simulink model "QuadCopter_2"  (R2018a)
settings: Solver=VariableStepAuto  StartTime=0.0  StopTime=60  MaxStep=0.1  RelTol=1e-3
values from neighbouring files (symbols this model uses):
  d = 2.4*10^-3    (= 0.0024)    [ScrValBackup.m]    (also in corke_plot.m = quad.d)
  dx0 = 0    [ScrValBackup.m]
  dy0 = 0    [ScrValBackup.m]
  dz0 = 0    [ScrValBackup.m]
  g = 9.81    [ScrValBackup.m]
  Ixx = 5.9*10-3    (= 56)    [ScrValBackup.m]    (also in quadrotorInitialValues.m)
  Iyy = 5.9*10-3    (= 56)    [ScrValBackup.m]    (also in quadrotorInitialValues.m)
  Izz = 1.16*10-3    (= 8.6)    [ScrValBackup.m]    (also in quadrotorInitialValues.m)
  K_lin = [   15.6000,    0.0000,    7.9000,    0.0000,         0 ... (first row only)    [ScrValBackup.m]
  kr = 0.1    [ScrValBackup.m]
  kt = 0.1    [ScrValBackup.m]
  l = 0.255    [ScrValBackup.m]
  m = 0.5    [ScrValBackup.m]
  p0 = 0    [ScrValBackup.m]
  phi0 = 0    [ScrValBackup.m]
  psi0 = 0.1    [ScrValBackup.m]
  q0 = 0    [ScrValBackup.m]
  r0 = 0.1177    [ScrValBackup.m]
  theta0 = 0    [ScrValBackup.m]
  x0 = 1    [ScrValBackup.m]    (also in corke_dynamics.m = init; corke_plot.m = [])
  x_coeff = A^-1*x_constr    [ScrValBackup.m]
  xd = 1    [ScrValBackup.m]
  y0 = 1    [ScrValBackup.m]
  y_coeff = A^-1*y_constr    [ScrValBackup.m]
  yd = 1    [ScrValBackup.m]
  z0 = 1    [ScrValBackup.m]
  z_coeff = A^-1*z_constr    [ScrValBackup.m]
  zd = 5    [ScrValBackup.m]
libraries: simulink x3, aerolibutil x1
settings Model: Creator=blue_orangotan  LastModifiedBy=giuseppe
settings SolverCC: ZeroCrossAlgorithm=Adaptive
settings DebuggingCC: MaxConsecutiveZCsMsg=warning  MaskedZcDiagnostic=none

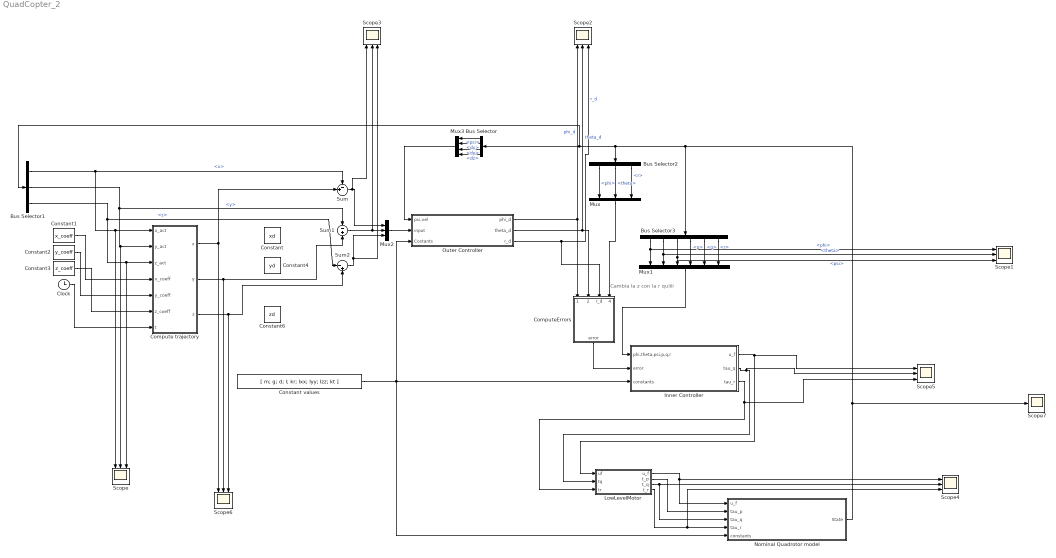
== system QuadCopter_2 ==
  note: Cambia la z con la r quiiii
  Bus Selector : BusSelector  OutputSignals=psi,dx,dy,dz
  Bus Selector1 : BusSelector  OutputSignals=x,y,z
  Bus Selector2 : BusSelector  OutputSignals=phi,theta,r
  Bus Selector3 : BusSelector  OutputSignals=phi,theta,psi,p,q,r
  Clock : Clock
  Compute trajectory : MATLAB Function  TreatAsAtomicUnit=on
  "ComputeErrors " : Subsystem
  Constant : Constant  Value=xd
  Constant values : Constant  Value=[ m; g; d; l; kr; Ixx; Iyy; Izz; kt ]
  Constant1 : Constant  Value=x_coeff
  Constant2 : Constant  Value=y_coeff
  Constant3 : Constant  Value=z_coeff
  Constant4 : Constant  Value=yd
  Constant6 : Constant  Value=zd
  "Inner Controller " : Subsystem
  LowLevelMotor : Subsystem
  Mux : Mux  Inputs=3
  Mux1 : Mux  Inputs=6
  Mux2 : Mux  Inputs=3
  Mux3 : Mux
  Nominal Quadrotor model : Subsystem
  "Outer Controller " : Subsystem
  Scope{,1..6} (7 alike) : Scope  NumInputPorts=3
  Scope7 : Scope
  Sum : Sum  Inputs=-+|
  Sum1 : Sum  Inputs=-+
  Sum2 : Sum  Inputs=|-+
  wires:
  Nominal Quadrotor model/1(State) -> Scope7/1, Bus Selector/1, Bus Selector1/1, Bus Selector2/1, Bus Selector3/1
  Constant values/1 -> "Inner Controller "/3(constants), Nominal Quadrotor model/5(constants), "Outer Controller "/3(Costants)
  Constant1/1 -> Compute trajectory/4(x_coeff)
  Constant2/1 -> Compute trajectory/5(y_coeff)
  Constant3/1 -> Compute trajectory/6(z_coeff)
  Clock/1 -> Compute trajectory/7(t)
  Bus Selector1/1 -> Sum/1, Compute trajectory/1(x_act), Scope/1  "<x>"
  Bus Selector1/2 -> Scope/2, Compute trajectory/2(y_act), Sum1/1  "<y>"
  Bus Selector1/3 -> Scope/3, Compute trajectory/3(z_act), Sum2/1  "<z>"
  "ComputeErrors "/1(error) -> "Inner Controller "/2(error)
  Bus Selector2/1 -> Mux/1  "<phi>"
  Bus Selector2/2 -> Mux/2  "<theta>"
  Bus Selector2/3 -> Mux/3  "<r>"
  Mux/1 -> "ComputeErrors "/4(Curr_values)
  Bus Selector3/1 -> Mux1/1, Scope1/1  "<phi>"
  Bus Selector3/2 -> Mux1/2, Scope1/2  "<theta>"
  Bus Selector3/3 -> Scope1/3, Mux1/3  "<psi>"
  Bus Selector3/4 -> Mux1/4  "<p>"
  Bus Selector3/5 -> Mux1/5  "<q>"
  Bus Selector3/6 -> Mux1/6  "<r>"
  Mux1/1 -> "Inner Controller "/1(phi,theta,psi,p,q,r)
  "Inner Controller "/1(u_f) -> Scope5/1, LowLevelMotor/1(uf)
  "Inner Controller "/2(tau_q) -> Scope5/2, LowLevelMotor/2("tq ")
  "Inner Controller "/3(tau_r) -> Scope5/3, LowLevelMotor/3(tr)
  LowLevelMotor/1(u_f) -> Scope4/1, Nominal Quadrotor model/1(u_f)
  LowLevelMotor/2(t_p) -> Nominal Quadrotor model/2(tau_p)
  LowLevelMotor/3(t_q) -> Scope4/2, Nominal Quadrotor model/3(tau_q)
  LowLevelMotor/4(t_r) -> Scope4/3, Nominal Quadrotor model/4(tau_r)
  "Outer Controller "/1("phi_d ") -> "ComputeErrors "/1(phi_d), Scope2/1  "phi_d"
  "Outer Controller "/2(theta_d) -> "ComputeErrors "/2(theta_d), Scope2/2  "theta_d"
  Sum/1 -> Scope3/1, Mux2/1
  Sum1/1 -> Mux2/2, Scope3/2
  Sum2/1 -> Scope3/3, Mux2/3
  Mux2/1 -> "Outer Controller "/2(input)
  "Outer Controller "/3(r_d) -> "ComputeErrors "/3(r_d), Scope2/3  "r_d"
  Compute trajectory/2(y) -> Sum1/2, Scope6/2
  Compute trajectory/1(x) -> Sum/2, Scope6/1
  Compute trajectory/3(z) -> Sum2/2, Scope6/3
  Bus Selector/1 -> Mux3/1  "<psi>"
  Bus Selector/2 -> Mux3/2  "<dx>"
  Bus Selector/3 -> Mux3/3  "<dy>"
  Bus Selector/4 -> Mux3/4  "<dz>"
  Mux3/1 -> "Outer Controller "/1(psi,vel)

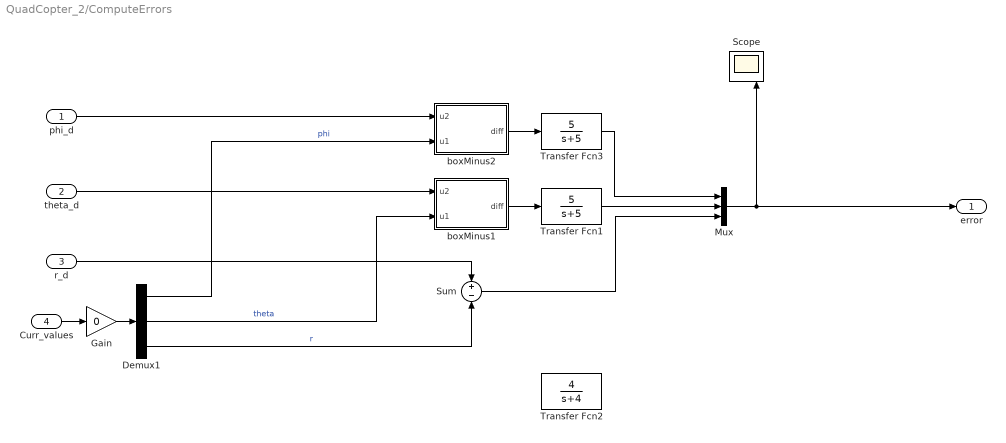
== system QuadCopter_2/ComputeErrors  ==
  phi_d : Inport
  theta_d : Inport  Port=2
  r_d : Inport  Port=3
  Curr_values : Inport  Port=4
  Demux1 : Demux  Outputs=3
  Gain : Gain  Gain=0
  Mux : Mux  Inputs=3
  Scope : Scope  NumInputPorts=3
  Sum : Sum  Inputs=+-
  Transfer Fcn1 : TransferFcn  Numerator=[5]  Denominator=[1 5]
  Transfer Fcn2 : TransferFcn  Numerator=[4]  Denominator=[1 4]
  Transfer Fcn3 : TransferFcn  Numerator=[5]  Denominator=[1 5]
  boxMinus1 : MATLAB Function  TreatAsAtomicUnit=on
  boxMinus2 : MATLAB Function  TreatAsAtomicUnit=on
  error : Outport
  wires:
  phi_d/1 -> boxMinus2/1(u2)
  Demux1/1 -> boxMinus2/2(u1)  "phi"
  theta_d/1 -> boxMinus1/1(u2)
  Demux1/2 -> boxMinus1/2(u1)  "theta"
  r_d/1 -> Sum/1
  Demux1/3 -> Sum/2  "r"
  Mux/1 -> error/1, Scope/3
  Sum/1 -> Mux/3
  boxMinus2/1(diff) -> Transfer Fcn3/1
  boxMinus1/1(diff) -> Transfer Fcn1/1
  Transfer Fcn3/1 -> Mux/1
  Transfer Fcn1/1 -> Mux/2
  Curr_values/1 -> Gain/1
  Gain/1 -> Demux1/1

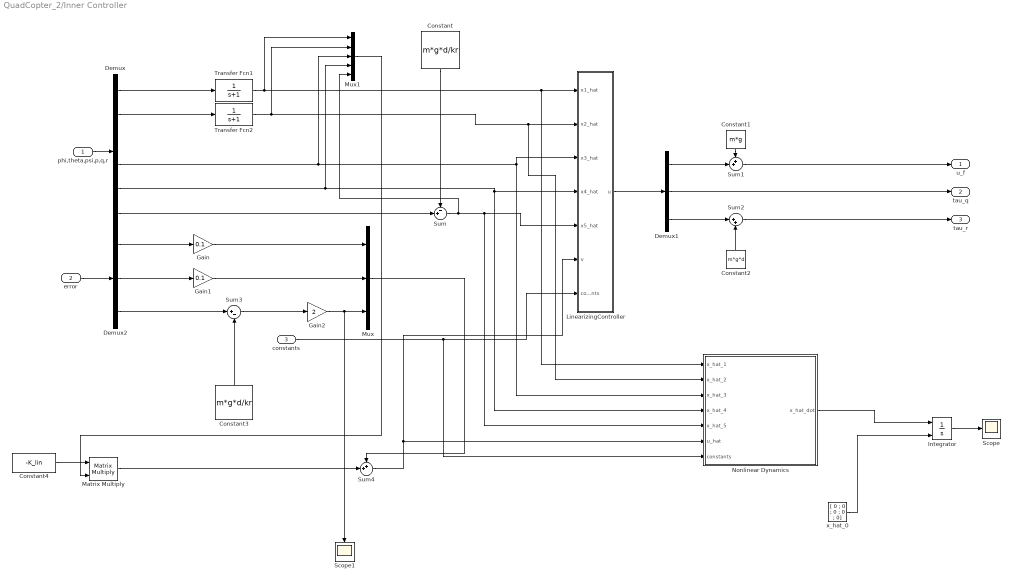
== system QuadCopter_2/Inner Controller  ==
  phi,theta,psi,p,q,r : Inport
  error : Inport  Port=2
  constants : Inport  Port=3
  Constant : Constant  Value=m*g*d/kr
  Constant1 : Constant  Value=m*g
  Constant2 : Constant  Value=m*g*d
  Constant3 : Constant  Value=m*g*d/kr
  Constant4 : Constant  Value=-K_lin
  Demux : Demux  Outputs=6
  Demux1 : Demux  Outputs=3
  Demux2 : Demux  Outputs=3
  Gain : Gain  Gain=0.1
  Gain1 : Gain  Gain=0.1
  Gain2 : Gain  Gain=2
  Integrator : Integrator  InitialConditionSource=external
  LinearizingController : MATLAB Function  TreatAsAtomicUnit=on
  Matrix Multiply : Product  Multiplication=Matrix(*)
  Mux : Mux  Inputs=3
  Mux1 : Mux  Inputs=5
  "Nonlinear Dynamics " : MATLAB Function  TreatAsAtomicUnit=on
  Scope : Scope
  Scope1 : Scope
  Sum : Sum  Inputs=-+|
  Sum1 : Sum  Inputs=++|
  Sum2 : Sum  Inputs=|++
  Sum3 : Sum  Inputs=|+-
  Sum4 : Sum  Inputs=++|
  Transfer Fcn1 : TransferFcn  Denominator=[1 1]
  Transfer Fcn2 : TransferFcn  Denominator=[1 1]
  x_hat_0 : Constant  Value=[ 0 ; 0 ; 0 ; 0 ; 0]
  u_f : Outport
  tau_q : Outport  Port=2
  tau_r : Outport  Port=3
  wires:
  phi,theta,psi,p,q,r/1 -> Demux/1
  Demux/1 -> Transfer Fcn1/1
  Demux/2 -> Transfer Fcn2/1
  Demux/4 -> Mux1/3, LinearizingController/3(x3_hat), "Nonlinear Dynamics "/3(x_hat_3)
  Demux/5 -> Mux1/4, "Nonlinear Dynamics "/4(x_hat_4), LinearizingController/4(x4_hat)
  "Nonlinear Dynamics "/1(x_hat_dot) -> Integrator/1
  x_hat_0/1 -> Integrator/2
  Constant/1 -> Sum/1
  Sum/1 -> Mux1/5, "Nonlinear Dynamics "/5(x_hat_5), LinearizingController/5(x5_hat)
  Demux1/3 -> Sum2/1
  Demux1/1 -> Sum1/2
  Constant1/1 -> Sum1/1
  Sum1/1 -> u_f/1
  Demux1/2 -> tau_q/1
  Constant2/1 -> Sum2/2
  Sum2/1 -> tau_r/1
  LinearizingController/1(u) -> Demux1/1
  Integrator/1 -> Scope/1
  constants/1 -> "Nonlinear Dynamics "/7(constants), LinearizingController/7(constants)
  Demux/6 -> Sum/2
  error/1 -> Demux2/1
  Constant3/1 -> Sum3/2
  Sum3/1 -> Gain2/1
  Transfer Fcn1/1 -> Mux1/1, "Nonlinear Dynamics "/1(x_hat_1), LinearizingController/1(x1_hat)
  Transfer Fcn2/1 -> Mux1/2, "Nonlinear Dynamics "/2(x_hat_2), LinearizingController/2(x2_hat)
  Demux2/1 -> Gain/1
  Demux2/2 -> Gain1/1
  Constant4/1 -> Matrix Multiply/1
  Mux1/1 -> Matrix Multiply/2
  Matrix Multiply/1 -> Sum4/2
  Mux/1 -> Sum4/1
  Sum4/1 -> "Nonlinear Dynamics "/6(u_hat), LinearizingController/6(v)
  Gain/1 -> Mux/1
  Gain1/1 -> Mux/2
  Demux2/3 -> Sum3/1
  Gain2/1 -> Mux/3, Scope1/1

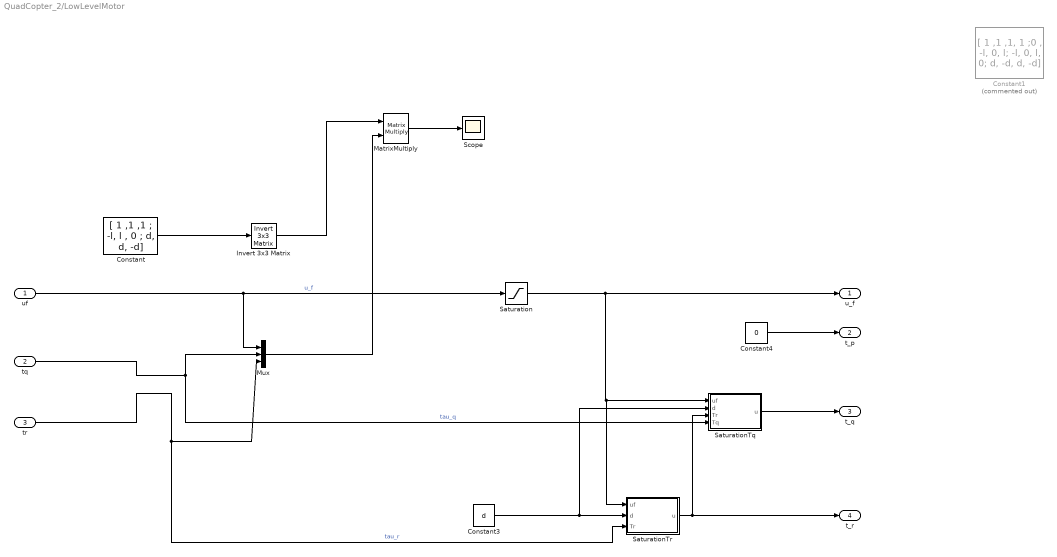
== system QuadCopter_2/LowLevelMotor ==
  uf : Inport
  "tq " : Inport  Port=2
  tr : Inport  Port=3
  Constant : Constant  Value=[ 1 ,1 ,1 ; -l, l , 0 ; d, d, -d]
  Constant1 : Constant  Commented=on  Value="[ 1 ,1 ,1, 1 ;0 , -l, 0, l;  -l, 0, l, 0; d, -d, d, -d]"
  Constant3 : Constant  Value=d
  Constant4 : Constant  Value=0
  Invert 3x3 Matrix : aerolibutil/Invert  3x3 Matrix
  MatrixMultiply : Product  Multiplication=Matrix(*)
  Mux : Mux  Inputs=3
  Saturation : Saturate  UpperLimit=15
  SaturationTq : MATLAB Function  TreatAsAtomicUnit=on
  SaturationTr : MATLAB Function  TreatAsAtomicUnit=on
  Scope : Scope
  u_f : Outport
  t_p : Outport  Port=2
  t_q : Outport  Port=3
  t_r : Outport  Port=4
  wires:
  "tq "/1 -> SaturationTq/4(Tq), Mux/2  "tau_q"
  tr/1 -> Mux/3, SaturationTr/3(Tr)  "tau_r"
  uf/1 -> Mux/1, Saturation/1  "u_f"
  Constant/1 -> Invert 3x3 Matrix/1
  Constant4/1 -> t_p/1
  Constant3/1 -> SaturationTq/2(d), SaturationTr/2(d)
  SaturationTr/1(u) -> SaturationTq/3(Tr), t_r/1
  SaturationTq/1(u) -> t_q/1
  Invert 3x3 Matrix/1 -> MatrixMultiply/1
  Saturation/1 -> SaturationTr/1(uf), SaturationTq/1(uf), u_f/1
  Mux/1 -> MatrixMultiply/2
  MatrixMultiply/1 -> Scope/1

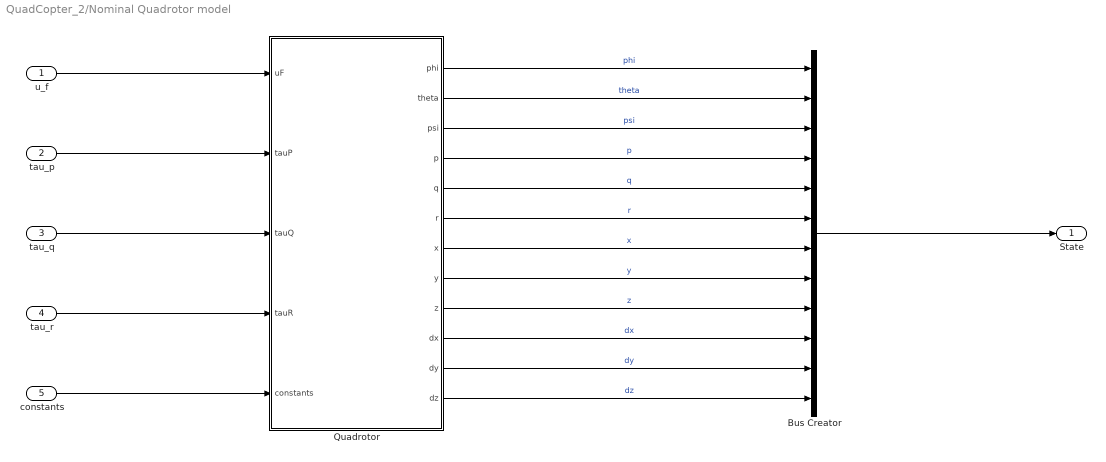
== system QuadCopter_2/Nominal Quadrotor model ==
  u_f : Inport
  tau_p : Inport  Port=2
  tau_q : Inport  Port=3
  tau_r : Inport  Port=4
  constants : Inport  Port=5
  Bus Creator : BusCreator  Inputs=12
  "Quadrotor " : Subsystem
  State : Outport
  wires:
  u_f/1 -> "Quadrotor "/1(uF)
  tau_q/1 -> "Quadrotor "/3(tauQ)
  tau_r/1 -> "Quadrotor "/4(tauR)
  constants/1 -> "Quadrotor "/5(constants)
  tau_p/1 -> "Quadrotor "/2(tauP)
  "Quadrotor "/1(phi) -> Bus Creator/1  "phi"
  "Quadrotor "/2(theta) -> Bus Creator/2  "theta"
  "Quadrotor "/3(psi) -> Bus Creator/3  "psi"
  "Quadrotor "/4(p) -> Bus Creator/4  "p"
  "Quadrotor "/5(q) -> Bus Creator/5  "q"
  "Quadrotor "/6(r) -> Bus Creator/6  "r"
  "Quadrotor "/7(x) -> Bus Creator/7  "x"
  "Quadrotor "/8(y) -> Bus Creator/8  "y"
  "Quadrotor "/9(z) -> Bus Creator/9  "z"
  Bus Creator/1 -> State/1
  "Quadrotor "/10(dx) -> Bus Creator/10  "dx"
  "Quadrotor "/11(dy) -> Bus Creator/11  "dy"
  "Quadrotor "/12(dz) -> Bus Creator/12  "dz"

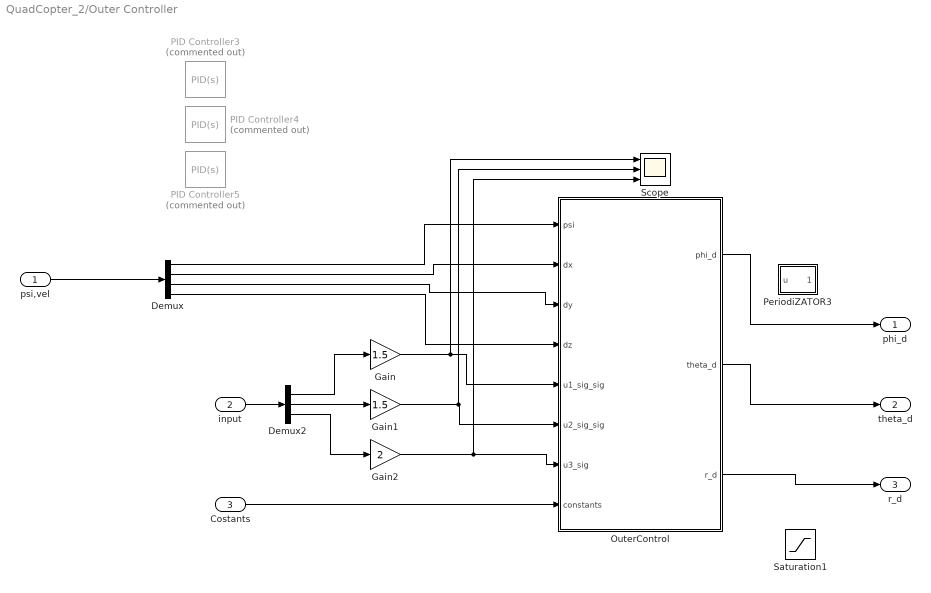
== system QuadCopter_2/Outer Controller  ==
  psi,vel : Inport  SampleTime=0.1
  input : Inport  Port=2
  Costants : Inport  Port=3
  Demux : Demux
  Demux2 : Demux  Outputs=3
  Gain : Gain  Gain=1.5
  Gain1 : Gain  Gain=1.5
  Gain2 : Gain  Gain=2
  OuterControl : MATLAB Function  TreatAsAtomicUnit=on
  PID Controller3 : simulink/Continuous/PID Controller  Commented=on  Controller=PID  TimeDomain=Continuous-time  SampleTime=-1  IntegratorMethod=Forward Euler  FilterMethod=Forward Euler  Form=Parallel  UseFilter=on  ControllerParametersSource=internal  P=-3.31812549008861e-05  I=-2.04327645124417e-11  D=-11.9723513961423  N=0.0120629646409386  InitialConditionSource=internal  InitialConditionForIntegrator=0  InitialConditionForFilter=0  ExternalReset=none  LimitOutput=off  UpperSaturationLimit=inf  LowerSaturationLimit=-inf  LinearizeAsGain=on  AntiWindupMode=none  Kb=1  TrackingMode=off  Kt=1  PParamMin=[]  PParamMax=[]  IParamMin=[]  IParamMax=[]  DParamMin=[]  DParamMax=[]  NParamMin=[]  NParamMax=[]  KbParamMin=[]  KbParamMax=[]  KtParamMin=[]  KtParamMax=[]  POutMin=[]  POutMax=[]  IOutMin=[]  IOutMax=[]  DOutMin=[]  DOutMax=[]  NOutMin=[]  NOutMax=[]  KbOutMin=[]  KbOutMax=[]  KtOutMin=[]  KtOutMax=[]  IntegratorOutMin=[]  IntegratorOutMax=[]  FilterOutMin=[]  FilterOutMax=[]  SumOutMin=[]  SumOutMax=[]  SumI1OutMin=[]  SumI1OutMax=[]  SumI2OutMin=[]  SumI2OutMax=[]  SumI3OutMin=[]  SumI3OutMax=[]  SumDOutMin=[]  SumDOutMax=[]  SaturationOutMin=[]  SaturationOutMax=[]  IntegratorContinuousStateAttributes=''  IntegratorStateMustResolveToSignalObject=off  IntegratorRTWStateStorageClass=Auto  FilterContinuousStateAttributes=''  FilterStateMustResolveToSignalObject=off  FilterRTWStateStorageClass=Auto  DifferentiatorICPrevScaledInput=0  DifferentiatorOutMin=[]  DifferentiatorOutMax=[]  FilterDiffOutCoefMin=[]  FilterDiffOutCoefMax=[]  SumDenOutMin=[]  SumDenOutMax=[]  SumNumOutMin=[]  SumNumOutMax=[]  ReciprocalOutMin=[]  ReciprocalOutMax=[]  DivideOutMin=[]  DivideOutMax=[]  TunerSelectOption=Transfer Function Based (PID Tuner App)
  PID Controller4 : simulink/Continuous/PID Controller  Commented=on  Controller=PID  TimeDomain=Continuous-time  SampleTime=-1  IntegratorMethod=Forward Euler  FilterMethod=Forward Euler  Form=Parallel  UseFilter=on  ControllerParametersSource=internal  P=-3.31812549008861e-05  I=-2.04327645124417e-11  D=-11.9723513961423  N=0.0120629646409386  InitialConditionSource=internal  InitialConditionForIntegrator=0  InitialConditionForFilter=0  ExternalReset=none  LimitOutput=off  UpperSaturationLimit=inf  LowerSaturationLimit=-inf  LinearizeAsGain=on  AntiWindupMode=none  Kb=1  TrackingMode=off  Kt=1  PParamMin=[]  PParamMax=[]  IParamMin=[]  IParamMax=[]  DParamMin=[]  DParamMax=[]  NParamMin=[]  NParamMax=[]  KbParamMin=[]  KbParamMax=[]  KtParamMin=[]  KtParamMax=[]  POutMin=[]  POutMax=[]  IOutMin=[]  IOutMax=[]  DOutMin=[]  DOutMax=[]  NOutMin=[]  NOutMax=[]  KbOutMin=[]  KbOutMax=[]  KtOutMin=[]  KtOutMax=[]  IntegratorOutMin=[]  IntegratorOutMax=[]  FilterOutMin=[]  FilterOutMax=[]  SumOutMin=[]  SumOutMax=[]  SumI1OutMin=[]  SumI1OutMax=[]  SumI2OutMin=[]  SumI2OutMax=[]  SumI3OutMin=[]  SumI3OutMax=[]  SumDOutMin=[]  SumDOutMax=[]  SaturationOutMin=[]  SaturationOutMax=[]  IntegratorContinuousStateAttributes=''  IntegratorStateMustResolveToSignalObject=off  IntegratorRTWStateStorageClass=Auto  FilterContinuousStateAttributes=''  FilterStateMustResolveToSignalObject=off  FilterRTWStateStorageClass=Auto  DifferentiatorICPrevScaledInput=0  DifferentiatorOutMin=[]  DifferentiatorOutMax=[]  FilterDiffOutCoefMin=[]  FilterDiffOutCoefMax=[]  SumDenOutMin=[]  SumDenOutMax=[]  SumNumOutMin=[]  SumNumOutMax=[]  ReciprocalOutMin=[]  ReciprocalOutMax=[]  DivideOutMin=[]  DivideOutMax=[]  TunerSelectOption=Transfer Function Based (PID Tuner App)
  PID Controller5 : simulink/Continuous/PID Controller  Commented=on  Controller=PID  TimeDomain=Continuous-time  SampleTime=-1  IntegratorMethod=Forward Euler  FilterMethod=Forward Euler  Form=Parallel  UseFilter=on  ControllerParametersSource=internal  P=-3.31812549008861e-05  I=-2.04327645124417e-11  D=-11.9723513961423  N=0.0120629646409386  InitialConditionSource=internal  InitialConditionForIntegrator=0  InitialConditionForFilter=0  ExternalReset=none  LimitOutput=off  UpperSaturationLimit=inf  LowerSaturationLimit=-inf  LinearizeAsGain=on  AntiWindupMode=none  Kb=1  TrackingMode=off  Kt=1  PParamMin=[]  PParamMax=[]  IParamMin=[]  IParamMax=[]  DParamMin=[]  DParamMax=[]  NParamMin=[]  NParamMax=[]  KbParamMin=[]  KbParamMax=[]  KtParamMin=[]  KtParamMax=[]  POutMin=[]  POutMax=[]  IOutMin=[]  IOutMax=[]  DOutMin=[]  DOutMax=[]  NOutMin=[]  NOutMax=[]  KbOutMin=[]  KbOutMax=[]  KtOutMin=[]  KtOutMax=[]  IntegratorOutMin=[]  IntegratorOutMax=[]  FilterOutMin=[]  FilterOutMax=[]  SumOutMin=[]  SumOutMax=[]  SumI1OutMin=[]  SumI1OutMax=[]  SumI2OutMin=[]  SumI2OutMax=[]  SumI3OutMin=[]  SumI3OutMax=[]  SumDOutMin=[]  SumDOutMax=[]  SaturationOutMin=[]  SaturationOutMax=[]  IntegratorContinuousStateAttributes=''  IntegratorStateMustResolveToSignalObject=off  IntegratorRTWStateStorageClass=Auto  FilterContinuousStateAttributes=''  FilterStateMustResolveToSignalObject=off  FilterRTWStateStorageClass=Auto  DifferentiatorICPrevScaledInput=0  DifferentiatorOutMin=[]  DifferentiatorOutMax=[]  FilterDiffOutCoefMin=[]  FilterDiffOutCoefMax=[]  SumDenOutMin=[]  SumDenOutMax=[]  SumNumOutMin=[]  SumNumOutMax=[]  ReciprocalOutMin=[]  ReciprocalOutMax=[]  DivideOutMin=[]  DivideOutMax=[]  TunerSelectOption=Transfer Function Based (PID Tuner App)
  PeriodiZATOR3 : MATLAB Function  TreatAsAtomicUnit=on
  Saturation1 : Saturate  UpperLimit=5  LowerLimit=0
  Scope : Scope  NumInputPorts=3
  "phi_d " : Outport
  theta_d : Outport  Port=2
  r_d : Outport  Port=3
  wires:
  Costants/1 -> OuterControl/8(constants)
  input/1 -> Demux2/1
  OuterControl/3(r_d) -> r_d/1
  Demux2/1 -> Gain/1
  Demux2/2 -> Gain1/1
  Demux2/3 -> Gain2/1
  Gain/1 -> Scope/1, OuterControl/5(u1_sig_sig)
  Gain1/1 -> Scope/2, OuterControl/6(u2_sig_sig)
  Gain2/1 -> Scope/3, OuterControl/7(u3_sig)
  OuterControl/1(phi_d) -> "phi_d "/1
  OuterControl/2(theta_d) -> theta_d/1
  psi,vel/1 -> Demux/1
  Demux/1 -> OuterControl/1(psi)
  Demux/2 -> OuterControl/2(dx)
  Demux/3 -> OuterControl/3(dy)
  Demux/4 -> OuterControl/4(dz)

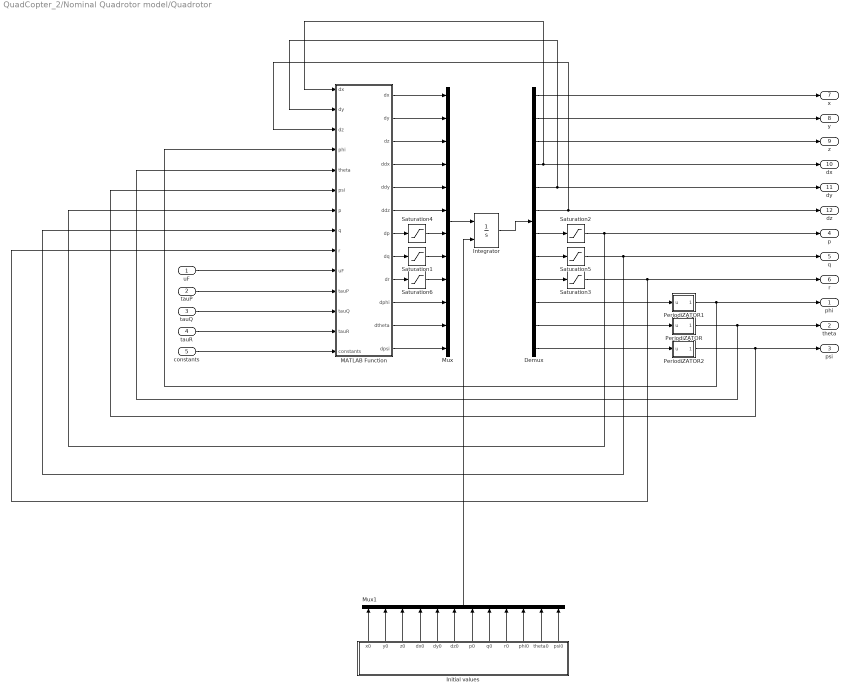
== system QuadCopter_2/Nominal Quadrotor model/Quadrotor  ==
  uF : Inport
  tauP : Inport  Port=2
  tauQ : Inport  Port=3
  tauR : Inport  Port=4
  constants : Inport  Port=5
  Demux : Demux  Outputs=12
  "Initial values " : Subsystem
  Integrator : Integrator  InitialConditionSource=external
  MATLAB Function : MATLAB Function  TreatAsAtomicUnit=on
  Mux : Mux  Inputs=12
  Mux1 : Mux  Inputs=12
  PeriodiZATOR : MATLAB Function  TreatAsAtomicUnit=on
  PeriodiZATOR1 : MATLAB Function  TreatAsAtomicUnit=on
  PeriodiZATOR2 : MATLAB Function  TreatAsAtomicUnit=on
  Saturation1 : Saturate
  Saturation2 : Saturate  UpperLimit=4  LowerLimit=-4
  Saturation3 : Saturate  UpperLimit=6  LowerLimit=0
  Saturation4 : Saturate
  Saturation5 : Saturate  UpperLimit=4  LowerLimit=-4
  Saturation6 : Saturate
  phi : Outport
  theta : Outport  Port=2
  psi : Outport  Port=3
  p : Outport  Port=4
  q : Outport  Port=5
  r : Outport  Port=6
  x : Outport  Port=7
  y : Outport  Port=8
  z : Outport  Port=9
  dx : Outport  Port=10
  dy : Outport  Port=11
  dz : Outport  Port=12
  wires:
  uF/1 -> MATLAB Function/10(uF)
  tauP/1 -> MATLAB Function/11(tauP)
  tauQ/1 -> MATLAB Function/12(tauQ)
  tauR/1 -> MATLAB Function/13(tauR)
  PeriodiZATOR/1(angle) -> MATLAB Function/5(theta), theta/1
  PeriodiZATOR1/1(angle) -> MATLAB Function/4(phi), phi/1
  PeriodiZATOR2/1(angle) -> MATLAB Function/6(psi), psi/1
  constants/1 -> MATLAB Function/14(constants)
  MATLAB Function/1(dx) -> Mux/1
  MATLAB Function/2(dy) -> Mux/2
  MATLAB Function/3(dz) -> Mux/3
  MATLAB Function/4(ddx) -> Mux/4
  MATLAB Function/5(ddy) -> Mux/5
  MATLAB Function/6(ddz) -> Mux/6
  MATLAB Function/7(dp) -> Saturation4/1
  MATLAB Function/8(dq) -> Saturation1/1
  MATLAB Function/9(dr) -> Saturation6/1
  MATLAB Function/10(dphi) -> Mux/10
  MATLAB Function/11(dtheta) -> Mux/11
  MATLAB Function/12(dpsi) -> Mux/12
  Mux/1 -> Integrator/1
  "Initial values "/1(x0) -> Mux1/1
  "Initial values "/2(y0) -> Mux1/2
  "Initial values "/3(z0) -> Mux1/3
  "Initial values "/4(dx0) -> Mux1/4
  "Initial values "/5(dy0) -> Mux1/5
  "Initial values "/6(dz0) -> Mux1/6
  "Initial values "/7(p0) -> Mux1/7
  "Initial values "/8(q0) -> Mux1/8
  "Initial values "/9(r0) -> Mux1/9
  "Initial values "/10(phi0) -> Mux1/10
  "Initial values "/11(theta0) -> Mux1/11
  "Initial values "/12(psi0) -> Mux1/12
  Mux1/1 -> Integrator/2
  Integrator/1 -> Demux/1
  Demux/1 -> x/1
  Demux/2 -> y/1
  Demux/3 -> z/1
  Demux/5 -> dy/1, MATLAB Function/2("dy ")
  Demux/6 -> dz/1, MATLAB Function/3("dz ")
  Demux/10 -> PeriodiZATOR1/1(u)
  Demux/11 -> PeriodiZATOR/1(u)
  Demux/12 -> PeriodiZATOR2/1(u)
  Demux/9 -> Saturation3/1
  Demux/7 -> Saturation2/1
  Demux/8 -> Saturation5/1
  Saturation3/1 -> r/1, MATLAB Function/9(r)
  Saturation4/1 -> Mux/7
  Saturation1/1 -> Mux/8
  Saturation2/1 -> p/1, MATLAB Function/7(p)
  Saturation5/1 -> q/1, MATLAB Function/8(q)
  Saturation6/1 -> Mux/9
  Demux/4 -> dx/1, MATLAB Function/1("dx ")

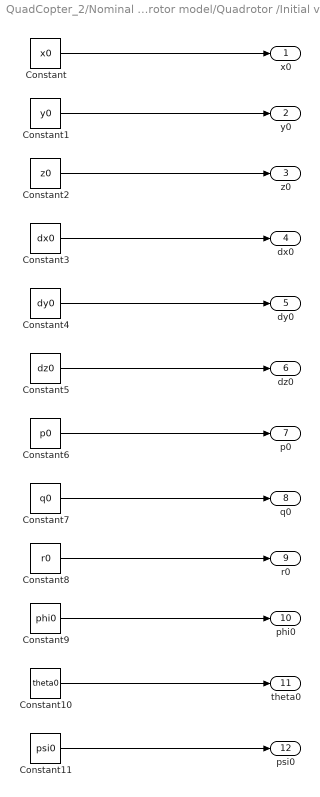
== system QuadCopter_2/Nominal Quadrotor model/Quadrotor /Initial values  ==
  Constant : Constant  Value=x0
  Constant1 : Constant  Value=y0
  Constant10 : Constant  Value=theta0
  Constant11 : Constant  Value=psi0
  Constant2 : Constant  Value=z0
  Constant3 : Constant  Value=dx0
  Constant4 : Constant  Value=dy0
  Constant5 : Constant  Value=dz0
  Constant6 : Constant  Value=p0
  Constant7 : Constant  Value=q0
  Constant8 : Constant  Value=r0
  Constant9 : Constant  Value=phi0
  x0 : Outport
  y0 : Outport  Port=2
  z0 : Outport  Port=3
  dx0 : Outport  Port=4
  dy0 : Outport  Port=5
  dz0 : Outport  Port=6
  p0 : Outport  Port=7
  q0 : Outport  Port=8
  r0 : Outport  Port=9
  phi0 : Outport  Port=10
  theta0 : Outport  Port=11
  psi0 : Outport  Port=12
  wires:
  Constant/1 -> x0/1
  Constant1/1 -> y0/1
  Constant2/1 -> z0/1
  Constant3/1 -> dx0/1
  Constant4/1 -> dy0/1
  Constant5/1 -> dz0/1
  Constant6/1 -> p0/1
  Constant7/1 -> q0/1
  Constant8/1 -> r0/1
  Constant9/1 -> phi0/1
  Constant10/1 -> theta0/1
  Constant11/1 -> psi0/1

== matlab function QuadCopter_2/Inner Controller /LinearizingController ==
  data: x1_hat input; u output; x2_hat input; x3_hat input; x4_hat input; x5_hat input; v input; constants input
function u = fcn(x1_hat,x2_hat,x3_hat,x4_hat,x5_hat, v, constants)

m= constants(1,1);
g= constants(2,1);
d= constants(3,1);
l= constants(4,1);
kr= constants(5,1);
Ixx= constants(6,1);
Iyy= constants(7,1);
Izz= constants(8,1);

alfa = zeros(3,1);

%% Non-robust feedback-linearation

alfa(1,1) = (2*Ixx*((kr*x3_hat - x4_hat*(x5_hat + (d*g*m)/kr)*(Ixx - Izz))/Ixx + (sin(x1_hat)*tan(x2_hat)*(x5_hat + (d*g*m)/kr) - x4_hat*cos(x1_hat)*tan(x2_hat))*(x3_hat + cos(x1_hat)*tan(x2_hat)*(x5_hat + (d*g*m)/kr) + x4_hat*sin(x1_hat)*tan(x2_hat)) + (sin(x1_hat)*(x5_hat + (d*g*m)/kr) - x4_hat*cos(x1_hat))*(cos(x1_hat)*(x5_hat + (d*g*m)/kr)*(tan(x2_hat)^2 + 1) + x4_hat*sin(x1_hat)*(tan(x2_hat)^2 + 1)) + (sin(x1_hat)*tan(x2_hat)*(kr*x4_hat + x3_hat*(x5_hat + (d*g*m)/kr)*(Ixx - Izz)))/Ixx + (kr*x5_hat*cos(x1_hat)*tan(x2_hat))/Izz))/l - (2*Ixx*sin(x1_hat)*tan(x2_hat)*((cos(x1_hat)*(x5_hat + (d*g*m)/kr) + x4_hat*sin(x1_hat))*(x3_hat + cos(x1_hat)*tan(x2_hat)*(x5_hat + (d*g*m)/kr) + x4_hat*sin(x1_hat)*tan(x2_hat)) + (cos(x1_hat)*(kr*x4_hat + x3_hat*(x5_hat + (d*g*m)/kr)*(Ixx - Izz)))/Ixx - (kr*x5_hat*sin(x1_hat))/Izz))/(l*cos(x1_hat)) - (kr*x5_hat*(2*Ixx*d*cos(x1_hat)^2*tan(x2_hat) - Izz*l*cos(x1_hat) + 2*Ixx*d*sin(x1_hat)^2*tan(x2_hat)))/(Izz*d*l*cos(x1_hat));
alfa(2,1) = (Ixx*((cos(x1_hat)*(x5_hat + (d*g*m)/kr) + x4_hat*sin(x1_hat))*(x3_hat + cos(x1_hat)*tan(x2_hat)*(x5_hat + (d*g*m)/kr) + x4_hat*sin(x1_hat)*tan(x2_hat)) + (cos(x1_hat)*(kr*x4_hat + x3_hat*(x5_hat + (d*g*m)/kr)*(Ixx - Izz)))/Ixx - (kr*x5_hat*sin(x1_hat))/Izz))/cos(x1_hat) + (Ixx*kr*x5_hat*sin(x1_hat))/(Izz*cos(x1_hat));
alfa(3,1) = kr*x5_hat;


beta =  [
         (2*Ixx)/l, -(2*Ixx*sin(x1_hat)*sin(x2_hat))/(l*cos(x1_hat)*cos(x2_hat)), -(2*Ixx*d*sin(x2_hat)-Izz*l*cos(x1_hat)*cos(x2_hat))/(d*l*cos(x1_hat)*cos(x2_hat));
         0,                                              Ixx/cos(x1_hat),                                                        (Ixx*sin(x1_hat))/cos(x1_hat);
         0,                                                            0,                                                                                  Izz];

%% Robust feedback linearization

% alfa(1,1) = x1_hat*((d*g*m*((2*Ixx*((d*g*m)/kr + (d*g*m*(Ixx - Izz))/(Ixx*kr)))/l + (2*kr*sin(x1_hat)*tan(x2_hat))/(l*cos(x1_hat))))/kr - (2*Ixx*d^2*g^2*m^2)/(kr^2*l)) - (sin(x1_hat)*(x5_hat + (d*g*m)/kr) - x4_hat*cos(x1_hat))*((2*Ixx*((d*g*m)/kr + (d*g*m*(Ixx - Izz))/(Ixx*kr)))/l + (2*kr*sin(x1_hat)*tan(x2_hat))/(l*cos(x1_hat))) + x2_hat*((d*g*m*((2*kr)/l - (2*Ixx*sin(x1_hat)*tan(x2_hat)*((d*g*m)/kr + (d*g*m*(Ixx - Izz))/(Ixx*kr)))/(l*cos(x1_hat))))/kr + (2*Ixx*d^2*g^2*m^2*sin(x1_hat)*tan(x2_hat))/(kr^2*l*cos(x1_hat))) - ((2*kr)/l - (2*Ixx*sin(x1_hat)*tan(x2_hat)*((d*g*m)/kr + (d*g*m*(Ixx - Izz))/(Ixx*kr)))/(l*cos(x1_hat)))*(x3_hat + cos(x1_hat)*tan(x2_hat)*(x5_hat + (d*g*m)/kr) + x4_hat*sin(x1_hat)*tan(x2_hat)) + (2*Ixx*((kr*x3_hat - x4_hat*(x5_hat + (d*g*m)/kr)*(Ixx - Izz))/Ixx + (sin(x1_hat)*tan(x2_hat)*(x5_hat + (d*g*m)/kr) - x4_hat*cos(x1_hat)*tan(x2_hat))*(x3_hat + cos(x1_hat)*tan(x2_hat)*(x5_hat + (d*g*m)/kr) + x4_hat*sin(x1_hat)*tan(x2_hat)) + (sin(x1_hat)*(x5_hat + (d*g*m)/kr) - x4_hat*cos(x1_hat))*(cos(x1_hat)*(x5_hat + (d*g*m)/kr)*(tan(x2_hat)^2 + 1) + x4_hat*sin(x1_hat)*(tan(x2_hat)^2 + 1)) + (sin(x1_hat)*tan(x2_hat)*(kr*x4_hat + x3_hat*(x5_hat + (d*g*m)/kr)*(Ixx - Izz)))/Ixx + (kr*x5_hat*cos(x1_hat)*tan(x2_hat))/Izz))/l - (2*Ixx*sin(x1_hat)*tan(x2_hat)*((cos(x1_hat)*(x5_hat + (d*g*m)/kr) + x4_hat*sin(x1_hat))*(x3_hat + cos(x1_hat)*tan(x2_hat)*(x5_hat + (d*g*m)/kr) + x4_hat*sin(x1_hat)*tan(x2_hat)) + (cos(x1_hat)*(kr*x4_hat + x3_hat*(x5_hat + (d*g*m)/kr)*(Ixx - Izz)))/Ixx - (kr*x5_hat*sin(x1_hat))/Izz))/(l*cos(x1_hat));
% alfa(2,1) = (kr*x5_hat*sin(x1_hat) - kr*x4_hat*cos(x1_hat) + d*g*m*sin(x1_hat))/cos(x1_hat) + (Ixx*((cos(x1_hat)*(kr*x4_hat + (x3_hat*(kr*x5_hat + d*g*m)*(Ixx - Izz))/kr))/Ixx + ((kr*x5_hat*cos(x1_hat) + kr*x4_hat*sin(x1_hat) + d*g*m*cos(x1_hat))*(x3_hat + x4_hat*sin(x1_hat)*tan(x2_hat) + (cos(x1_hat)*tan(x2_hat)*(kr*x5_hat + d*g*m))/kr))/kr - (kr*x5_hat*sin(x1_hat))/Izz))/cos(x1_hat) - (d*g*m*x1_hat)/cos(x1_hat) - (d*g*m*(2*Ixx - Izz)*(x3_hat + x4_hat*sin(x1_hat)*tan(x2_hat) + (cos(x1_hat)*tan(x2_hat)*(kr*x5_hat + d*g*m))/kr))/(kr*cos(x1_hat)) + (d^2*g^2*m^2*x2_hat*(Ixx - Izz))/(kr^2*cos(x1_hat));
% alfa(3,1) = 0;
% 
% beta = [
%         1, -(2*sin(x1_hat)*sin(x2_hat))/(l*cos(x1_hat)*cos(x2_hat)), -(2*Ixx*sin(x2_hat))/(Izz*l*cos(x1_hat)*cos(x2_hat));
%         0,                                            1/cos(x1_hat),                  (Ixx*sin(x1_hat))/(Izz*cos(x1_hat));
%         0,                                                        0,                                                    1];
    
u = alfa + beta*v;

== matlab function QuadCopter_2/LowLevelMotor/SaturationTr ==
  data: uf input; u output; d input; Tr input
function u = fcn(uf, d, Tr)

if abs(Tr) > d*uf
    Tr = sign(Tr)*d*uf;
end

u = Tr;

== matlab function QuadCopter_2/Inner Controller /Nonlinear Dynamics  ==
  data: x_hat_1 input; x_hat_2 input; x_hat_3 input; x_hat_4 input; x_hat_5 input; x_hat_dot output; u_hat input; constants input
function x_hat_dot = fcn(x_hat_1,x_hat_2,x_hat_3,x_hat_4,x_hat_5,u_hat,constants)

m= constants(1,1);
g= constants(2,1);
d= constants(3,1);
l= constants(4,1);
kr= constants(5,1);
Ixx= constants(6,1);
Iyy= constants(7,1);
Izz= constants(8,1);

x_hat = [x_hat_1;
        x_hat_2;
        x_hat_3;
        x_hat_4;
        x_hat_5];

f = [
    x_hat(3,1)+x_hat(4,1)*sin(x_hat(1,1))*tan(x_hat(2,1)) + ( x_hat(5,1)+ m*g*d/kr)*cos(x_hat(1,1))*tan(x_hat(2,1));
    x_hat(4,1)*cos(x_hat(1,1))- (x_hat(5,1)+ m*g*d/kr)*sin(x_hat(1,1)) ;
    1/Ixx*( -kr*x_hat(3,1)- x_hat(4,1)*(x_hat(5,1)+ m*g*d/kr)*(Izz - Ixx));
    1/Iyy*( -kr*x_hat(4,1)- x_hat(3,1)*(x_hat(5,1)+ m*g*d/kr)*(Ixx - Izz));
    1/Izz*(-kr* x_hat(5,1));    
    ];
G = [
    0 , 0 , 0;
    0,  0 , 0;
    l/(2*Ixx), 0 , -l/(2*d*Ixx)
    0,  1/Iyy  , 0 ;
    0 ,  0   ,  1/Izz;
    ];

    
x_hat_dot = f + G*u_hat;

== matlab function QuadCopter_2/LowLevelMotor/SaturationTq ==
  data: uf input; u output; d input; Tr input; Tq input
function u = fcn(uf, d, Tr, Tq)

if abs(Tq) > (0.5*(uf+Tr/d))
    Tq = sign(Tq)*(0.5*(uf+Tr/d));
end

u = Tq;

== matlab function QuadCopter_2/ComputeErrors /boxMinus1 ==
  data: u2 input; diff output; u1 input
function diff = fcn(u2, u1)

R2 = [cos(u2) -sin(u2);
      sin(u2) cos(u2)];

R1 = [cos(-u1) -sin(-u1);
      sin(-u1) cos(-u1)];

R = R2*R1;

diff = atan2(R(2,1), R(1,1));

== matlab function QuadCopter_2/ComputeErrors /boxMinus2 ==
  data: u2 input; diff output; u1 input
function diff = fcn(u2, u1)

R2 = [cos(u2) -sin(u2);
      sin(u2) cos(u2)];

R1 = [cos(-u1) -sin(-u1);
      sin(-u1) cos(-u1)];

R = R2*R1;

diff = atan2(R(2,1), R(1,1));

== matlab function QuadCopter_2/Compute trajectory ==
  data: x_act input; y_act input; z_act input; x_coeff input; x output; y_coeff input; z_coeff input; t input; y output; z output
function [x, y, z]  = fcn(x_act, y_act, z_act, x_coeff, y_coeff, z_coeff, t)

x_ = x_coeff(1)*t^3+x_coeff(2)*t^2+x_coeff(3)*t+x_coeff(4);
y_ = y_coeff(1)*t^3+y_coeff(2)*t^2+y_coeff(3)*t+y_coeff(4);
z_ = z_coeff(1)*t^3+z_coeff(2)*t^2+z_coeff(3)*t+z_coeff(4);

x_ddot = 6*x_coeff(1)*t+2*x_coeff(2);
y_ddot = 6*y_coeff(1)*t+2*y_coeff(2);
z_ddot = 6*z_coeff(1)*t+2*z_coeff(2);

u = zeros(3,1);

% u(1,1) = x_ddot + 100*(x_ - x_act);
% u(2,1) = y_ddot + 100*(y_ - y_act);
% u(3,1) = z_ddot + 100*(z_ - z_act);
x = x_;
y = y_;
z = z_;

== matlab function QuadCopter_2/Outer Controller /OuterControl ==
  data: psi input; dx input; dy input; dz input; phi_d output; u1_sig_sig input; u2_sig_sig input; u3_sig input; theta_d output; r_d output; constants input
function [phi_d , theta_d , r_d ] = fcn(psi, dx, dy, dz, u1_sig_sig, u2_sig_sig, u3_sig, constants)

m= constants(1,1);
g= constants(2,1);
d= constants(3,1);
l= constants(4,1);
kr= constants(5,1);
Ixx= constants(6,1);
Iyy= constants(7,1);
Izz= constants(8,1);
kt= constants(9,1);

R = [sin(psi), cos(psi);
    -cos(psi), sin(psi)];

u_sig_sig = [(u1_sig_sig+kt/m*dx) (u2_sig_sig+kt/m*dy)]';

u12 = R'*u_sig_sig;

u3_sig = u3_sig + g;

r_d = u3_sig*m*d/kr;
phi_d= u12(1)/u3_sig;
theta_d = u12(2)/u3_sig;

== matlab function QuadCopter_2/Nominal Quadrotor model/Quadrotor /MATLAB Function ==
  data: dx output; dy output; dz output; dx input; dy input; dz input; phi input; theta input; psi input; p input; q input; r input; uF input; ddx output; tauP input; tauQ input; tauR input; ddy output; ddz output; dp output; dq output; dr output; dphi output; dtheta output; dpsi output; constants input
function [dx,dy,dz,ddx,ddy,ddz,dp,dq,dr,dphi,dtheta,dpsi] = fcn(dx, dy, dz, phi, theta, psi, p, q, r, uF, tauP, tauQ, tauR, constants)

    m= constants(1,1);
    g= constants(2,1);
    d= constants(3,1);
    l= constants(4,1);
    kr= constants(5,1);
    Ixx= constants(6,1);
    Iyy= constants(7,1);
    Izz= constants(8,1);
    kt = constants(9,1);

    
    ddx = (1/m)*((cos(phi)*cos(psi)*sin(theta) + sin(phi)*sin(psi))*uF - kt*dx);
    
    ddy = (1/m)*((cos(phi)*sin(theta)*sin(psi) - cos(psi)*sin(phi))*uF - kt*dy);
    
    ddz = (1/m)*((cos(theta)*cos(phi))*uF - m*g - kt*dz);
    
%     dp = (1/Ixx)*(-kr*p - q*r*(Izz - Iyy) + tauP);

    dp = (1/Ixx)*(-kr*p - q*r*(Izz - Iyy) + l/2*(uF - tauR/d));
    
    dq = (1/Iyy)*(-kr*q - p*r*(Ixx - Izz) + tauQ);
    
    dr = (1/Izz)*(-kr*r - p*q*(Iyy - Ixx) + tauR);
    
%     dr = 1/Izz*(-kr*r + tauR);
    
    dphi = p + q*sin(phi)*tan(phi) + r*cos(phi)*tan(theta);
    
    dtheta = q*cos(phi) - r*sin(phi);
    
    dpsi = (1/cos(theta))*(q*sin(phi) + r*cos(phi));

== matlab function QuadCopter_2/Nominal Quadrotor model/Quadrotor /PeriodiZATOR ==
  data: u input; angle output
function angle = fcn(u)

y = sin(u);
x = cos(u);

% angle = mod(u, 2*pi)
angle = atan2(y,x);

== matlab function QuadCopter_2/Nominal Quadrotor model/Quadrotor /PeriodiZATOR1 ==
  data: u input; angle output
function angle = fcn(u)

y = sin(u);
x = cos(u);

% angle = mod(u, 2*pi)
angle = atan2(y,x);

== matlab function QuadCopter_2/Nominal Quadrotor model/Quadrotor /PeriodiZATOR2 ==
  data: u input; angle output
function angle = fcn(u)

y = sin(u);
x = cos(u);

% angle = mod(u, 2*pi);
angle = atan2(y,x);

== matlab function QuadCopter_2/Outer Controller /PeriodiZATOR3 ==
  data: u input; angle output
function angle = fcn(u)

y = sin(u);
x = cos(u);

% angle = mod(u, 2*pi);
angle = atan2(y,x);
